simulink model "MOT_CTRL_CTRL_FUN_004"  (R2025a)
settings: Solver=FixedStepAuto  StartTime=0.0  StopTime=10.0  FixedStep=1e-4  RelTol=1e-3
settings Model: DataDictionary=PIDControl.sldd  Creator=tecnicomcbti  LastModifiedBy=tecnicomcbti
settings SolverCC: ConcurrentTasks=on  AutoInsertRateTranBlk=on
settings DebuggingCC: UnderspecifiedInitializationDetection=Classic  MergeDetectMultiDrivingBlocksExec=none
settings ModelReferenceCC: PropagateSignalLabelsOutOfModel=off

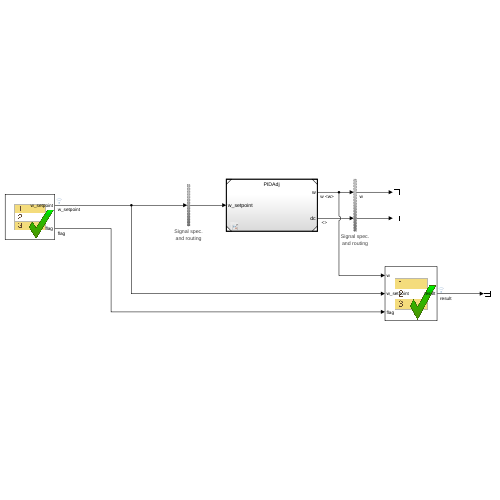
[thumbnail: Simulink's stored preview of the top-level diagram]
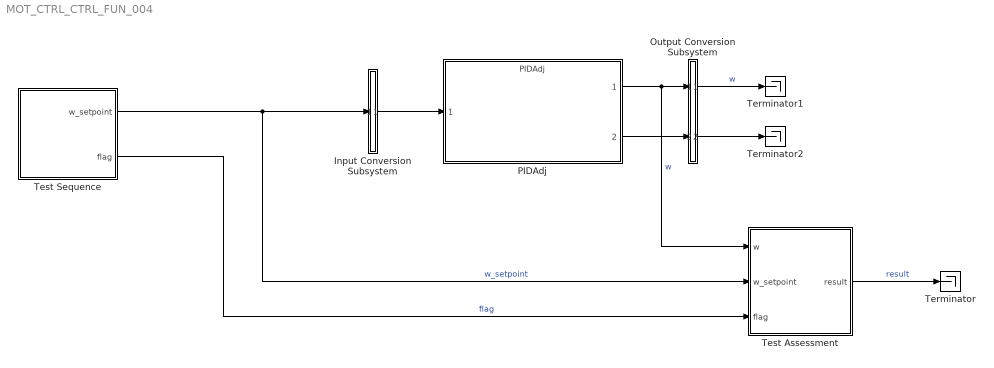
== system MOT_CTRL_CTRL_FUN_004 ==
  Input Conversion Subsystem : Subsystem  Tag=__SLT_ICS__  Description=|
      | Signal spec.
      | and routing
      settings: AttributesFormatString=%<Description>
  Output Conversion Subsystem : Subsystem  Tag=__SLT_OCS__  Description=|
      | Signal spec.
      | and routing
      settings: AttributesFormatString=%<Description>
  PIDAdj : ModelReference  ModelNameDialog=PIDAdj  SimulationMode=Normal  ModelReferenceVersion=1.17
  Terminator : Terminator
  Terminator1 : Terminator
  Terminator2 : Terminator
  Test Assessment : Test Sequence  TreatAsAtomicUnit=on
  Test Sequence : Test Sequence  TreatAsAtomicUnit=on
  wires:
  Output Conversion Subsystem/1(Outport_1) -> Terminator1/1  "w"
  Output Conversion Subsystem/2(Outport_2) -> Terminator2/1
  Input Conversion Subsystem/1(Outport_1) -> PIDAdj/1
  PIDAdj/1 -> Test Assessment/1(w), Output Conversion Subsystem/1(Inport_1)  "w"
  PIDAdj/2 -> Output Conversion Subsystem/2(Inport_2)
  Test Sequence/2(flag) -> Test Assessment/3(flag)  "flag"
  Test Sequence/1(w_setpoint) -> Input Conversion Subsystem/1(Inport_1), Test Assessment/2(w_setpoint)  "w_setpoint"
  Test Assessment/1(result) -> Terminator/1  "result"

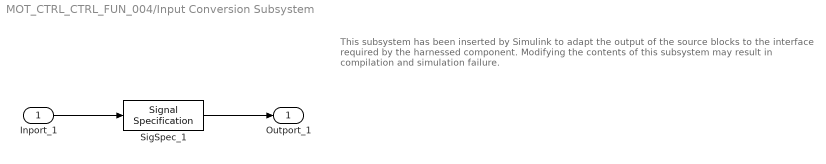
== system MOT_CTRL_CTRL_FUN_004/Input Conversion Subsystem ==
  note: This subsystem has been inserted by Simulink to adapt the output of the source blocks to the interface required by the harnessed component.
      |  Modifying the contents of this subsystem may result in compilation and simulation failure.
  Inport_1 : Inport
  SigSpec_1 : SignalSpecification  OutDataTypeStr=double  Dimensions=[1]  SampleTime=0.001
  Outport_1 : Outport
  wires:
  SigSpec_1/1 -> Outport_1/1
  Inport_1/1 -> SigSpec_1/1

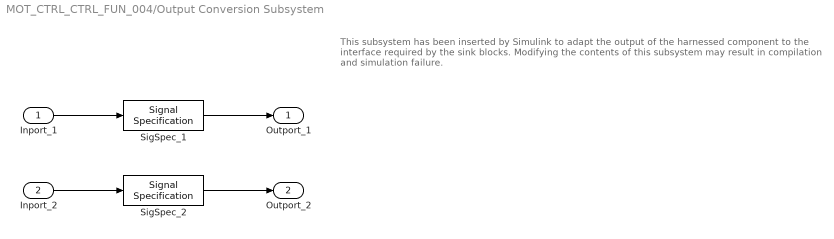
== system MOT_CTRL_CTRL_FUN_004/Output Conversion Subsystem ==
  note: This subsystem has been inserted by Simulink to adapt the output of the harnessed component to the interface required by the sink blocks.
      |  Modifying the contents of this subsystem may result in compilation and simulation failure.
  Inport_1 : Inport
  Inport_2 : Inport  Port=2
  SigSpec_1 : SignalSpecification  OutDataTypeStr=double  Dimensions=[1]
  SigSpec_2 : SignalSpecification  OutDataTypeStr=double  Dimensions=[1]  SampleTime=0.001
  Outport_1 : Outport
  Outport_2 : Outport  Port=2
  wires:
  Inport_1/1 -> SigSpec_1/1
  SigSpec_1/1 -> Outport_1/1
  Inport_2/1 -> SigSpec_2/1
  SigSpec_2/1 -> Outport_2/1

== stateflow chart MOT_CTRL_CTRL_FUN_004/Test Assessment ==
  state step_1
    state step_1_1
      if((w > 0.98*w_setpoint) && (w < 1.02*w_setpoint))
      result = true;
      else
      result = false;
      end
    state step_1_2
    (default) -> (junction 22)
    step_1 -> (junction 22)
    (junction 22) -> (junction 23) [order 1] : [(flag)
        | ]
    (junction 23) -> step_1_1 [order 1] : [~in(step_1.step_1_1)]
    (junction 22) -> (junction 31) [order 2]
    (junction 23) -> (junction 26) [order 2]
    (junction 31) -> (junction 32)
    (junction 32) -> step_1_2 [order 1] : [~in(step_1.step_1_2)]
    (junction 32) -> (junction 35) [order 2]
  (default) -> step_1
  data: w input; w_setpoint input; flag input boolean; result output boolean

== stateflow chart MOT_CTRL_CTRL_FUN_004/Test Sequence ==
  state Start
    flag = false;
    w_setpoint = 0;
  state Degrau
    flag = false;
    w_setpoint = 5100*pi/30;
  state Resposta_estacionaria
    flag = true;
    w_setpoint = 5100*pi/30;
  (default) -> Start
  Start -> Degrau : [
      | after(1,sec)
      | ]
  Degrau -> Resposta_estacionaria : [
      | after(settling_time,sec)
      | ]
  data: w_setpoint output; flag output boolean; settling_time constant double =5
